simulink model "VxSpdEsti0725"  (R2022b)
settings: Solver=VariableStepAuto  StartTime=0.0  StopTime=10.0  RelTol=1e-3
undefined symbols (not defined in the file): DiscIntNeverNeededParam, Ldwf, Ldwr, Q, Qa, R, Ra, thr1, thr2, thr3, thr4, thr5, TrqRquRate
libraries: simulink x45
settings Model: Creator=12045  LastModifiedBy=12045

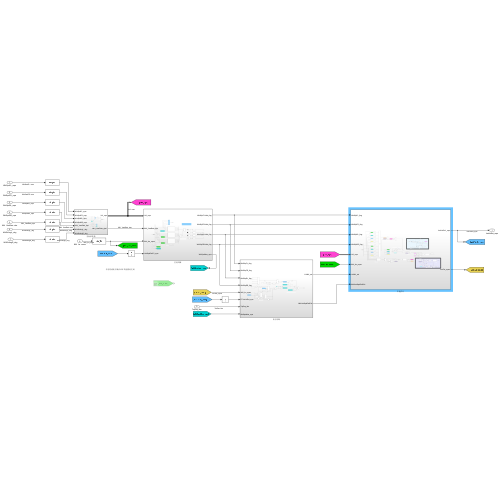
[thumbnail: Simulink's stored preview of the top-level diagram]
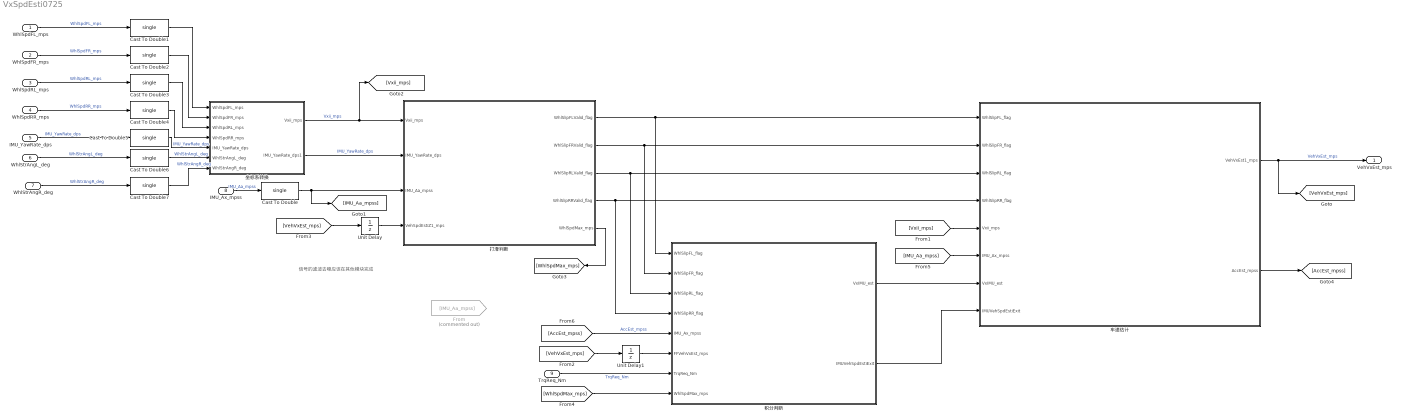
== system VxSpdEsti0725 ==
  note: 信号的滤波去噪应该在其他模块完成
  WhlSpdFL_mps : Inport
  WhlSpdFR_mps : Inport  Port=2
  WhlSpdRL_mps : Inport  Port=3
  WhlSpdRR_mps : Inport  Port=4
  IMU_YawRate_dps : Inport  Port=5
  WhlStrAngL_deg : Inport  Port=6
  WhlStrAngR_deg : Inport  Port=7
  IMU_Ax_mpss : Inport  Port=8
  TrqReq_Nm : Inport  Port=9
  Cast To Double{,1..7} (8 alike) : DataTypeConversion  OutDataTypeStr=single  SaturateOnIntegerOverflow=off  RndMeth=Floor
  From : From  Commented=on  GotoTag=IMU_Aa_mpss
  Unit Delay : UnitDelay  SampleTime=-1  HasFrameUpgradeWarning=on
  Unit Delay1 : UnitDelay  SampleTime=-1  HasFrameUpgradeWarning=on
  坐标系转换 : Subsystem
  打滑判断 : Subsystem
  积分判断 : Subsystem
  车速估计 : Subsystem
  VehVxEst_mps : Outport
  wires:
  [AccEst_mpss] -> 积分判断/5(IMU_Ax_mpss)  "AccEst_mpss"
  [Vxii_mps] -> 车速估计/5(Vxii_mps)
  Unit Delay/1 -> 打滑判断/4(VehSpdEstiZ1_mps)
  打滑判断/3(WhlSlipRLValid_flag) -> 积分判断/3(WhlSlipRL_flag), 车速估计/3(WhlSlipRL_flag)
  WhlSpdFR_mps/1 -> Cast To Double2/1  "WhlSpdFR_mps"
  打滑判断/5(WhlSpdMax_mps) -> [WhlSpdMax_mps]
  Cast To Double4/1 -> 坐标系转换/4(WhlSpdRR_mps)
  Cast To Double7/1 -> 坐标系转换/7(WhlStrAngR_deg)  "WhlStrAngR_deg"
  Unit Delay1/1 -> 积分判断/6(FFVehVxEst_mps)
  Cast To Double6/1 -> 坐标系转换/6(WhlStrAngL_deg)  "WhlStrAngL_deg"
  Cast To Double/1 -> [IMU_Aa_mpss], 打滑判断/3(IMU_Aa_mpss)
  Cast To Double3/1 -> 坐标系转换/3(WhlSpdRL_mps)
  WhlSpdFL_mps/1 -> Cast To Double1/1  "WhlSpdFL_mps"
  [VehVxEst_mps] -> Unit Delay/1
  TrqReq_Nm/1 -> 积分判断/7(TrqReq_Nm)  "TrqReq_Nm"
  [IMU_Aa_mpss] -> 车速估计/6(IMU_Ax_mpss)
  Cast To Double1/1 -> 坐标系转换/1(WhlSpdFL_mps)
  WhlSpdRR_mps/1 -> Cast To Double4/1  "WhlSpdRR_mps"
  打滑判断/2(WhlSlipFRValid_flag) -> 积分判断/2(WhlSlipFR_flag), 车速估计/2(WhlSlipFR_flag)
  Cast To Double2/1 -> 坐标系转换/2(WhlSpdFR_mps)
  [WhlSpdMax_mps] -> 积分判断/8(WhlSpdMax_mps)
  WhlSpdRL_mps/1 -> Cast To Double3/1  "WhlSpdRL_mps"
  车速估计/2(AccEst_mpss) -> [AccEst_mpss]
  积分判断/1(VxIMU_est) -> 车速估计/7(VxIMU_est)
  Cast To Double5/1 -> 坐标系转换/5(IMU_YawRate_dps)  "IMU_YawRate_dps"
  打滑判断/1(WhlSlipFLValid_flag) -> 积分判断/1(WhlSlipFL_flag), 车速估计/1(WhlSlipFL_flag)
  打滑判断/4(WhlSlipRRValid_flag) -> 积分判断/4(WhlSlipRR_flag), 车速估计/4(WhlSlipRR_flag)
  积分判断/2(IMUVehSpdEstiExit) -> 车速估计/8(IMUVehSpdEstiExit)
  [VehVxEst_mps] -> Unit Delay1/1
  IMU_Ax_mpss/1 -> Cast To Double/1  "IMU_Aa_mpss"
  WhlStrAngL_deg/1 -> Cast To Double6/1  "WhlStrAngL_deg"
  车速估计/1(VehVxEst1_mps) -> [VehVxEst_mps], VehVxEst_mps/1  "VehVxEst_mps"
  坐标系转换/2(IMU_YawRate_dps1) -> 打滑判断/2(IMU_YawRate_dps)  "IMU_YawRate_dps"
  IMU_YawRate_dps/1 -> Cast To Double5/1  "IMU_YawRate_dps"
  WhlStrAngR_deg/1 -> Cast To Double7/1  "WhlStrAngR_deg"
  坐标系转换/1(Vxii_mps) -> [Vxii_mps], 打滑判断/1(Vxii_mps)  "Vxii_mps"

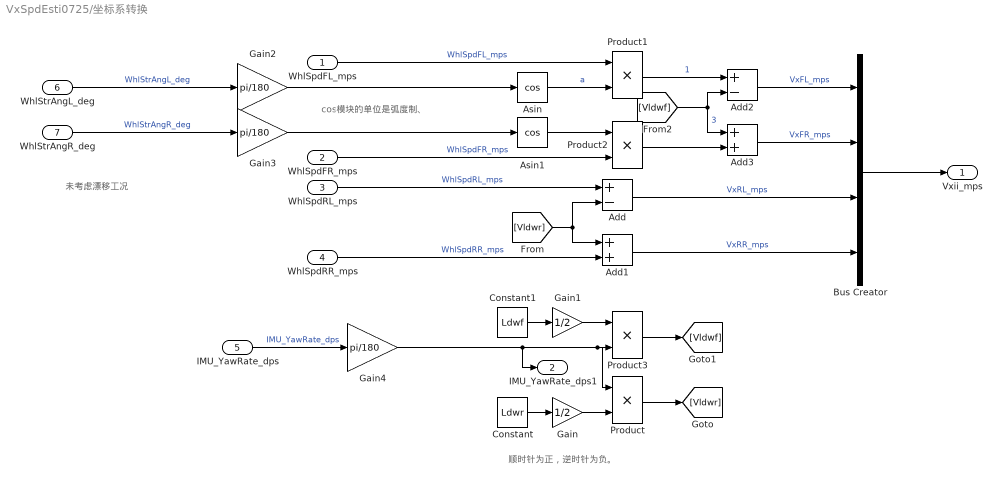
== system VxSpdEsti0725/坐标系转换 ==
  note: cos模块的单位是弧度制、
  note: 未考虑漂移工况
  note: 顺时针为正，逆时针为负。
  WhlSpdFL_mps : Inport
  WhlSpdFR_mps : Inport  Port=2
  WhlSpdRL_mps : Inport  Port=3
  WhlSpdRR_mps : Inport  Port=4
  IMU_YawRate_dps : Inport  Port=5
  WhlStrAngL_deg : Inport  Port=6
  WhlStrAngR_deg : Inport  Port=7
  Add : Sum  Inputs=+-
  Add1 : Sum
  Add2 : Sum  Inputs=+-
  Add3 : Sum
  Asin : Trigonometry  Operator=cos
  Asin1 : Trigonometry  Operator=cos
  Bus Creator : BusCreator  Inputs=4
  Constant : Constant  Value=Ldwr
  Constant1 : Constant  Value=Ldwf
  Gain : Gain  Gain=1/2
  Gain1 : Gain  Gain=1/2
  Gain2 : Gain  Gain=pi/180
  Gain3 : Gain  Gain=pi/180
  Gain4 : Gain  Gain=pi/180
  Product{,1..3} (4 alike) : Product
  Vxii_mps : Outport
  IMU_YawRate_dps1 : Outport  Port=2
  wires:
  Constant/1 -> Gain/1
  Gain/1 -> Product/2
  IMU_YawRate_dps/1 -> Gain4/1  "IMU_YawRate_dps"
  WhlSpdRL_mps/1 -> Add/1  "WhlSpdRL_mps"
  WhlSpdRR_mps/1 -> Add1/2  "WhlSpdRR_mps"
  Product/1 -> [Vldwr]
  [Vldwr] -> Add/2, Add1/1
  WhlSpdFL_mps/1 -> Product1/1  "WhlSpdFL_mps"
  WhlSpdFR_mps/1 -> Product2/2  "WhlSpdFR_mps"
  Constant1/1 -> Gain1/1
  Gain1/1 -> Product3/1
  Product3/1 -> [Vldwf]
  Product1/1 -> Add2/1  "1"
  [Vldwf] -> Add2/2, Add3/1  "3"
  Product2/1 -> Add3/2
  Add2/1 -> Bus Creator/1  "VxFL_mps"
  Add/1 -> Bus Creator/3  "VxRL_mps"
  Add3/1 -> Bus Creator/2  "VxFR_mps"
  Add1/1 -> Bus Creator/4  "VxRR_mps"
  Bus Creator/1 -> Vxii_mps/1
  Asin1/1 -> Product2/1
  WhlStrAngR_deg/1 -> Gain3/1  "WhlStrAngR_deg"
  WhlStrAngL_deg/1 -> Gain2/1  "WhlStrAngL_deg"
  Asin/1 -> Product1/2  "a"
  Gain2/1 -> Asin/1
  Gain3/1 -> Asin1/1
  Gain4/1 -> IMU_YawRate_dps1/1, Product/1, Product3/2

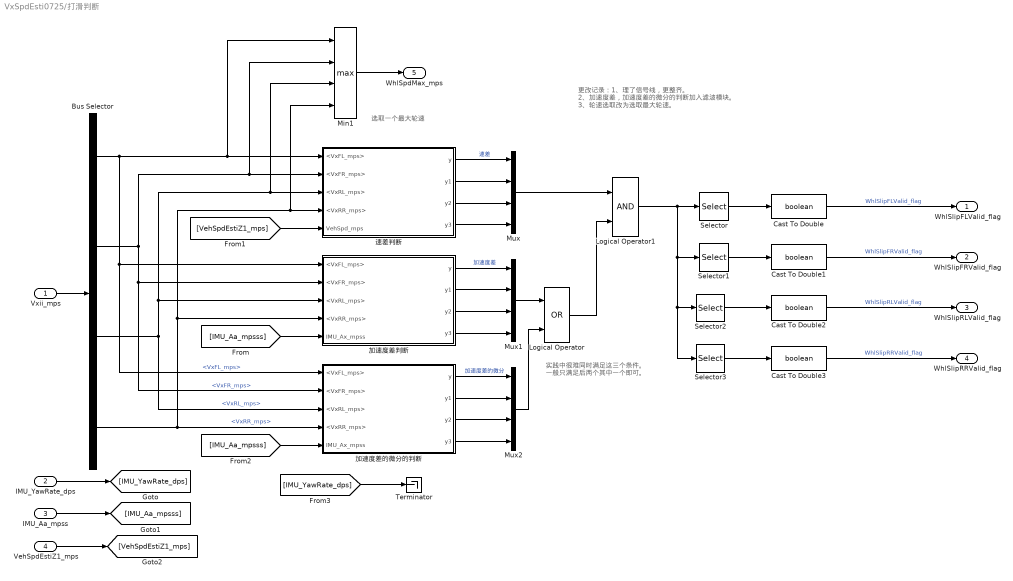
== system VxSpdEsti0725/打滑判断 ==
  note: 实践中很难同时满足这三个条件。
      | 一般只满足后两个其中一个即可。
  note: 更改记录：1、理了信号线，更整齐。
      | 2、加速度差，加速度差的微分的判断加入滤波模块。
      | 3、轮速选取改为选取最大轮速。
  note: 选取一个最大轮速
  Vxii_mps : Inport
  IMU_YawRate_dps : Inport  Port=2
  IMU_Aa_mpss : Inport  Port=3
  VehSpdEstiZ1_mps : Inport  Port=4
  Bus Selector : BusSelector  OutputSignals=VxFL_mps,VxFR_mps,VxRL_mps,VxRR_mps
  Cast To Double{,1..3} (4 alike) : DataTypeConversion  OutDataTypeStr=boolean  SaturateOnIntegerOverflow=off  RndMeth=Floor
  Logical Operator : Logic  Operator=OR  AllPortsSameDT=off  OutDataTypeStr=boolean
  Logical Operator1 : Logic  AllPortsSameDT=off  OutDataTypeStr=boolean
  Min1 : MinMax  Function=max  Inputs=4
  Mux : Mux
  Mux1 : Mux
  Mux2 : Mux
  Selector : Selector  InputPortWidth=4  IndexOptions=Index vector (dialog)  Indices=[1]  OutputSizes=1
  Selector1 : Selector  InputPortWidth=4  IndexOptions=Index vector (dialog)  Indices=[2]  OutputSizes=1
  Selector2 : Selector  InputPortWidth=4  IndexOptions=Index vector (dialog)  Indices=[3]  OutputSizes=1
  Selector3 : Selector  InputPortWidth=4  IndexOptions=Index vector (dialog)  Indices=[4]  OutputSizes=1
  Terminator : Terminator
  加速度差判断 : Subsystem
  加速度差的微分的判断 : Subsystem
  速差判断 : Subsystem
  WhlSlipFLValid_flag : Outport
  WhlSlipFRValid_flag : Outport  Port=2
  WhlSlipRLValid_flag : Outport  Port=3
  WhlSlipRRValid_flag : Outport  Port=4
  WhlSpdMax_mps : Outport  Port=5
  wires:
  Selector3/1 -> Cast To Double3/1
  Selector2/1 -> Cast To Double2/1
  [IMU_Aa_mpsss] -> 加速度差的微分的判断/5(IMU_Ax_mpss)
  [VehSpdEstiZ1_mps] -> 速差判断/5(VehSpd_mps)
  Bus Selector/3 -> 加速度差的微分的判断/3(<VxRL_mps>), 速差判断/3(<VxRL_mps>), Min1/3, 加速度差判断/3(<VxRL_mps>)  "<VxRL_mps>"
  Selector1/1 -> Cast To Double1/1
  [IMU_Aa_mpsss] -> 加速度差判断/5(IMU_Ax_mpss)
  Bus Selector/4 -> 加速度差判断/4(<VxRR_mps>), Min1/4, 速差判断/4(<VxRR_mps>), 加速度差的微分的判断/4(<VxRR_mps>)  "<VxRR_mps>"
  IMU_YawRate_dps/1 -> [IMU_YawRate_dps]
  Vxii_mps/1 -> Bus Selector/1
  Bus Selector/1 -> 加速度差的微分的判断/1(<VxFL_mps>), 加速度差判断/1(<VxFL_mps>), 速差判断/1(<VxFL_mps>), Min1/1  "<VxFL_mps>"
  VehSpdEstiZ1_mps/1 -> [VehSpdEstiZ1_mps]
  Selector/1 -> Cast To Double/1
  Bus Selector/2 -> 加速度差的微分的判断/2(<VxFR_mps>), 加速度差判断/2(<VxFR_mps>), 速差判断/2(<VxFR_mps>), Min1/2  "<VxFR_mps>"
  IMU_Aa_mpss/1 -> [IMU_Aa_mpsss]
  [IMU_YawRate_dps] -> Terminator/1
  Cast To Double/1 -> WhlSlipFLValid_flag/1  "WhlSlipFLValid_flag"
  Cast To Double1/1 -> WhlSlipFRValid_flag/1  "WhlSlipFRValid_flag"
  Cast To Double2/1 -> WhlSlipRLValid_flag/1  "WhlSlipRLValid_flag"
  Cast To Double3/1 -> WhlSlipRRValid_flag/1  "WhlSlipRRValid_flag"
  速差判断/1(y) -> Mux/1  "速差"
  速差判断/2(y1) -> Mux/2
  速差判断/3(y2) -> Mux/3
  速差判断/4(y3) -> Mux/4
  加速度差判断/1(y) -> Mux1/1  "加速度差"
  加速度差判断/2(y1) -> Mux1/2
  加速度差判断/3(y2) -> Mux1/3
  加速度差判断/4(y3) -> Mux1/4
  加速度差的微分的判断/1(y) -> Mux2/1  "加速度差的微分"
  加速度差的微分的判断/2(y1) -> Mux2/2
  加速度差的微分的判断/3(y2) -> Mux2/3
  加速度差的微分的判断/4(y3) -> Mux2/4
  Mux1/1 -> Logical Operator/1
  Mux2/1 -> Logical Operator/2
  Mux/1 -> Logical Operator1/1
  Logical Operator/1 -> Logical Operator1/2
  Logical Operator1/1 -> Selector3/1, Selector2/1, Selector1/1, Selector/1
  Min1/1 -> WhlSpdMax_mps/1

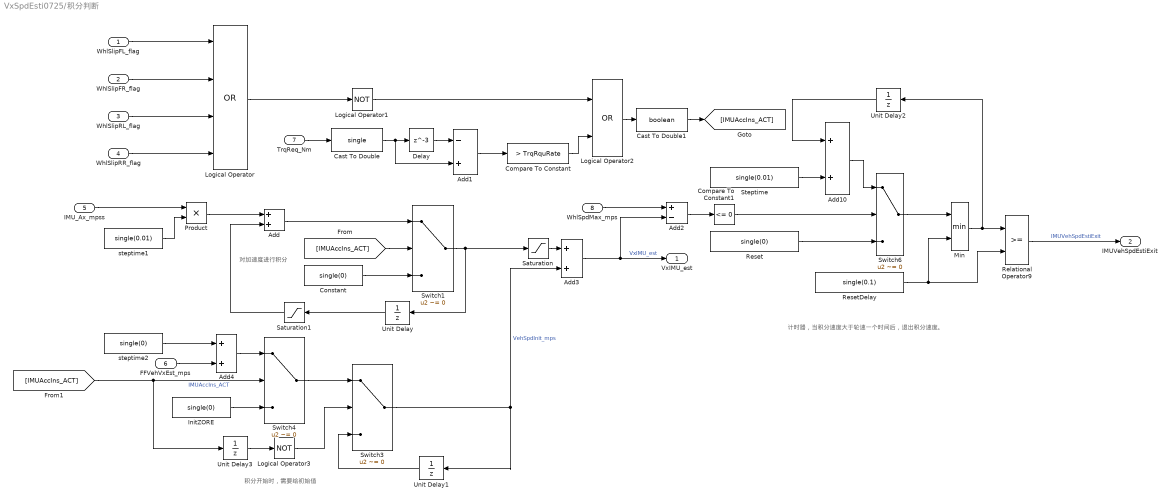
== system VxSpdEsti0725/积分判断 ==
  note: 对加速度进行积分
  note: 计时器，当积分速度大于轮速一个时间后，退出积分速度。
  note: 积分开始时，需要给初始值
  WhlSlipFL_flag : Inport
  WhlSlipFR_flag : Inport  Port=2
  WhlSlipRL_flag : Inport  Port=3
  WhlSlipRR_flag : Inport  Port=4
  IMU_Ax_mpss : Inport  Port=5
  FFVehVxEst_mps : Inport  Port=6
  TrqReq_Nm : Inport  Port=7
  WhlSpdMax_mps : Inport  Port=8
  Add{,3..4,10} (4 alike) : Sum
  Add1 : Sum  Inputs=-+
  Add2 : Sum  Inputs=+-
  Cast To Double : DataTypeConversion  OutDataTypeStr=single  SaturateOnIntegerOverflow=off  RndMeth=Floor
  Cast To Double1 : DataTypeConversion  OutDataTypeStr=boolean  SaturateOnIntegerOverflow=off  RndMeth=Floor
  Compare To Constant : simulink/Logic and Bit Operations/Compare To Constant  relop=>  const=TrqRquRate  OutDataTypeStr=boolean
  Compare To Constant1 : simulink/Logic and Bit Operations/Compare To Constant  relop=<=  const=0  OutDataTypeStr=boolean
  Constant : Constant  Value=single(0)
  Delay : Delay  DelayLength=3
  InitZORE : Constant  Value=single(0)
  Logical Operator : Logic  Operator=OR  Inputs=4  AllPortsSameDT=off  OutDataTypeStr=boolean
  Logical Operator1 : Logic  Operator=NOT  AllPortsSameDT=off  OutDataTypeStr=boolean
  Logical Operator2 : Logic  Operator=OR  AllPortsSameDT=off  OutDataTypeStr=boolean
  Logical Operator3 : Logic  Operator=NOT  AllPortsSameDT=off  OutDataTypeStr=boolean
  Min : MinMax  Inputs=2
  Product : Product
  Relational Operator9 : RelationalOperator  OutDataTypeStr=boolean  RndMeth=Simplest  InputSameDT=off
  Reset : Constant  Value=single(0)
  ResetDelay : Constant  Value=single(0.1)
  Saturation : Saturate  UpperLimit=200  LowerLimit=-10
  Saturation1 : Saturate  UpperLimit=200  LowerLimit=-10
  Steptime : Constant  Value=single(0.01)
  Switch{1,3..4,6} (4 alike) : Switch  Criteria=u2 ~= 0  SaturateOnIntegerOverflow=off  InputSameDT=off
  Unit Delay{,1..3} (4 alike) : UnitDelay  SampleTime=-1  HasFrameUpgradeWarning=on
  steptime1 : Constant  Value=single(0.01)
  steptime2 : Constant  Value=single(0)
  VxIMU_est : Outport
  IMUVehSpdEstiExit : Outport  Port=2
  wires:
  WhlSlipFL_flag/1 -> Logical Operator/1
  WhlSlipFR_flag/1 -> Logical Operator/2
  WhlSlipRL_flag/1 -> Logical Operator/3
  WhlSlipRR_flag/1 -> Logical Operator/4
  Logical Operator/1 -> Logical Operator1/1
  Unit Delay/1 -> Saturation1/1
  Add/1 -> Switch1/1
  Constant/1 -> Switch1/3
  Logical Operator1/1 -> Logical Operator2/1
  TrqReq_Nm/1 -> Cast To Double/1
  Delay/1 -> Add1/1
  Add1/1 -> Compare To Constant/1
  Compare To Constant/1 -> Logical Operator2/2
  [IMUAccIns_ACT] -> Switch1/2
  Logical Operator2/1 -> Cast To Double1/1
  Add2/1 -> Compare To Constant1/1
  WhlSpdMax_mps/1 -> Add2/1
  Saturation1/1 -> Add/2
  Product/1 -> Add/1
  IMU_Ax_mpss/1 -> Product/1
  steptime1/1 -> Product/2
  Saturation/1 -> Add3/1
  Add3/1 -> Add2/2, VxIMU_est/1  "VxIMU_est"
  Switch6/1 -> Min/1
  ResetDelay/1 -> Relational Operator9/2, Min/2
  Compare To Constant1/1 -> Switch6/2
  Add10/1 -> Switch6/1
  Steptime/1 -> Add10/2
  Min/1 -> Relational Operator9/1, Unit Delay2/1
  Reset/1 -> Switch6/3
  Unit Delay2/1 -> Add10/1
  Unit Delay3/1 -> Logical Operator3/1
  InitZORE/1 -> Switch4/3
  Logical Operator3/1 -> Switch3/2
  Switch3/1 -> Add3/2, Unit Delay1/1  "VehSpdInit_mps"
  Switch4/1 -> Switch3/1
  Cast To Double/1 -> Delay/1, Add1/2
  [IMUAccIns_ACT] -> Unit Delay3/1, Switch4/2  "IMUAccIns_ACT"
  Relational Operator9/1 -> IMUVehSpdEstiExit/1  "IMUVehSpdEstiExit"
  Cast To Double1/1 -> [IMUAccIns_ACT]
  Unit Delay1/1 -> Switch3/3
  Add4/1 -> Switch4/1
  FFVehVxEst_mps/1 -> Add4/2
  steptime2/1 -> Add4/1
  Switch1/1 -> Saturation/1, Unit Delay/1

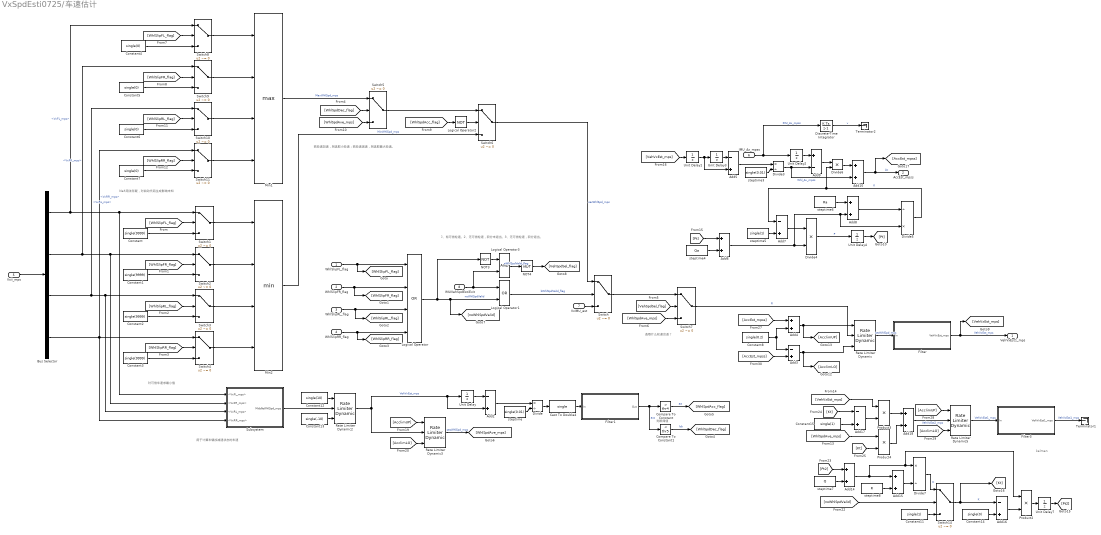
== system VxSpdEsti0725/车速估计 ==
  note: kalman
  note: 用于计算车辆加减速状态的车速
  note: 1、有可信轮速。2、无可信轮速，积分未退出。3、无可信轮速，积分退出。
  note: 选取什么轮速合适？
  note: 判断阈值
  note: 若轮速加速，则选取小轮速；若轮速减速，则选取最大轮速。
  note: NaN用法存疑，对自动代码生成影响未知
  note: 对可信车速求最小值
  WhlSlipFL_flag : Inport
  WhlSlipFR_flag : Inport  Port=2
  WhlSlipRL_flag : Inport  Port=3
  WhlSlipRR_flag : Inport  Port=4
  Vxii_mps : Inport  Port=5
  IMU_Ax_mpss : Inport  Port=6
  VxIMU_est : Inport  Port=7
  IMUVehSpdEstiExit : Inport  Port=8
  Add{4,6,8,10,14..15,18} (7 alike) : Sum
  Add{2..3,5,7,16..17} (6 alike) : Sum  Inputs=-+
  Add9 : Sum  Inputs=+-
  Bus Selector : BusSelector  OutputSignals=VxFL_mps,VxFR_mps,VxRL_mps,VxRR_mps
  Cast To Double4 : DataTypeConversion  OutDataTypeStr=single  SaturateOnIntegerOverflow=off  RndMeth=Floor
  Compare To Constant : simulink/Logic and Bit Operations/Compare To Constant  relop=>  const=thr4  OutDataTypeStr=boolean
  Compare To Constant1 : simulink/Logic and Bit Operations/Compare To Constant  relop=<  const=thr5  OutDataTypeStr=boolean
  Constant{,1..3} (4 alike) : Constant  Value=single(9999)
  Constant11 : Constant  Value=single(1)
  Constant12 : Constant  Value=single(10)
  Constant13 : Constant  Value=single(-10)
  Constant{4..7,14} (5 alike) : Constant  Value=single(0)
  Constant15 : Constant  Value=single(1)
  Constant8 : Constant  Value=single(0.2)
  Discrete-Time Integrator : DiscreteIntegrator  SampleTime=-1  ICPrevOutput=DiscIntNeverNeededParam  ICPrevScaledInput=DiscIntNeverNeededParam
  Divide : Product  Inputs=*/
  Divide3 : Product  Inputs=*/
  Divide4 : Product  Inputs=**
  Divide5 : Product  Inputs=/*
  Divide6 : Product  Inputs=**
  Divide7 : Product  Inputs=*/
  Filter : Subsystem
  Filter1 : Subsystem
  Filter3 : Subsystem
  Logical Operator : Logic  Operator=OR  Inputs=4  AllPortsSameDT=off  OutDataTypeStr=boolean
  Logical Operator1 : Logic  Operator=OR  AllPortsSameDT=off  OutDataTypeStr=boolean
  Logical Operator2 : Logic  Operator=NOT  AllPortsSameDT=off  OutDataTypeStr=boolean
  Logical Operator3 : Logic  AllPortsSameDT=off  OutDataTypeStr=boolean
  Min1 : MinMax  Function=max  Inputs=4
  Min2 : MinMax  Inputs=4
  NOT3 : Logic  Operator=NOT  AllPortsSameDT=off  OutDataTypeStr=boolean
  NOT4 : Logic  Operator=NOT  AllPortsSameDT=off  OutDataTypeStr=boolean
  Product2 : Product
  Product3 : Product
  Product4 : Product
  Rate Limiter Dynamic{,2..3,5} (4 alike) : simulink/Discontinuities/Rate Limiter Dynamic
  Subsystem : Subsystem
  Switch{,1..11,14} (13 alike) : Switch  Criteria=u2 ~= 0  SaturateOnIntegerOverflow=off  InputSameDT=off
  Terminator1 : Terminator
  Terminator2 : Terminator
  Unit Delay{,1..3,7} (5 alike) : UnitDelay  SampleTime=-1  HasFrameUpgradeWarning=on
  Unit Delay4 : UnitDelay  InitialCondition=0.01  SampleTime=-1  HasFrameUpgradeWarning=on
  steptime : Constant  Value=single(0.01)
  steptime3 : Constant  Value=single(0.01)
  steptime4 : Constant  Value=Qa
  steptime5 : Constant  Value=single(1)
  steptime6 : Constant  Value=Ra
  steptime7 : Constant  Value=Q
  steptime8 : Constant  Value=R
  VehVxEst1_mps : Outport
  AccEst_mpss : Outport  Port=2
  wires:
  Compare To Constant/1 -> [WhlSpdAcc_flag]  "aa"
  Vxii_mps/1 -> Bus Selector/1
  WhlSlipRR_flag/1 -> [WhlSlipRR_flag], Logical Operator/4
  Logical Operator3/1 -> NOT4/1  "aWhlSpdValid_flag"
  [VehSpdSel_flag] -> Switch7/2
  Logical Operator2/1 -> Switch6/2
  [WhlSlipFL_flag] -> Switch1/2
  Switch5/1 -> Switch6/1
  Constant/1 -> Switch1/3
  Compare To Constant1/1 -> [WhlSpdDec_flag]  "bb"
  Unit Delay/1 -> Add2/1
  [WhlSpdAve_mps] -> Switch5/3
  Filter1/1(Out) -> Compare To Constant1/1, Compare To Constant/1  "acc"
  Constant3/1 -> Switch4/3
  Logical Operator1/1 -> Switch/2  "bWhlSpdValid_flag"
  Switch4/1 -> Min2/4
  Constant2/1 -> Switch3/3
  [WhlSlipRR_flag] -> Switch4/2
  Switch1/1 -> Min2/1
  WhlSlipFR_flag/1 -> [WhlSlipFR_flag], Logical Operator/2
  [WhlSpdAcc_flag] -> Logical Operator2/1
  [WhlSlipRL_flag] -> Switch3/2
  Switch2/1 -> Min2/2
  Logical Operator/1 -> [noWhlSpdValid], Logical Operator1/2, NOT3/1  "noWhlSpdValid"
  WhlSlipFL_flag/1 -> [WhlSlipFL_flag], Logical Operator/1
  Constant1/1 -> Switch2/3
  Cast To Double4/1 -> Filter1/1(In)
  [WhlSpdDec_flag] -> Switch5/2
  [WhlSlipFR_flag] -> Switch2/2
  WhlSlipRL_flag/1 -> [WhlSlipRL_flag], Logical Operator/3
  Switch3/1 -> Min2/3
  [WhlSpdAve_mps] -> Switch7/3
  Add2/1 -> Divide/1
  Divide/1 -> Cast To Double4/1
  steptime/1 -> Divide/2
  Bus Selector/1 -> Switch8/1, Subsystem/1(<VxFL_mps>), Switch1/1  "<VxFL_mps>"
  Bus Selector/4 -> Subsystem/4(<VxRR_mps>), Switch11/1, Switch4/1  "<VxRR_mps>"
  [WhlSlipFR_flag] -> Switch9/2
  Bus Selector/2 -> Switch9/1, Subsystem/2(<VxFR_mps>), Switch2/1  "<VxFR_mps>"
  Constant5/1 -> Switch9/3
  Bus Selector/3 -> Switch10/1, Subsystem/3(<VxRL_mps>), Switch3/1  "<VxRL_mps>"
  [WhlSlipRL_flag] -> Switch10/2
  [WhlSlipRR_flag] -> Switch11/2
  Constant6/1 -> Switch10/3
  Constant7/1 -> Switch11/3
  Constant4/1 -> Switch8/3
  [WhlSlipFL_flag] -> Switch8/2
  Switch8/1 -> Min1/1
  Switch9/1 -> Min1/2
  Switch10/1 -> Min1/3
  Switch11/1 -> Min1/4
  Min1/1 -> Switch5/1  "MaxWhlSpd_mps"
  Subsystem/1(MiddleWhlSpd_mps) -> Rate Limiter Dynamic2/2
  Constant12/1 -> Rate Limiter Dynamic2/1
  Constant13/1 -> Rate Limiter Dynamic2/3
  Rate Limiter Dynamic2/1 -> Rate Limiter Dynamic3/2, Add2/2, Unit Delay/1  "VehVxEst_mps"
  Min2/1 -> Switch6/3  "MinWhlSpd_mps"
  IMUVehSpdEstiExit/1 -> Logical Operator3/2, Logical Operator1/1
  NOT3/1 -> Logical Operator3/1
  NOT4/1 -> [VehSpdSel_flag]
  Divide5/1 -> Add7/1, Divide6/2  "K"
  Unit Delay3/1 -> Add5/1
  steptime3/1 -> Divide3/2
  Add5/1 -> Divide3/1
  Unit Delay4/1 -> [Pt]
  [Pt] -> Add6/1
  steptime4/1 -> Add6/2
  Add6/1 -> Divide5/2, Add8/2, Divide4/2
  steptime5/1 -> Add7/2
  Add7/1 -> Divide4/1
  Divide4/1 -> Unit Delay4/1  "P"
  steptime6/1 -> Add8/1
  Add8/1 -> Divide5/1
  Divide3/1 -> Add10/2, Add9/2  "Whl_Ax_mpss"
  Add9/1 -> Divide6/1
  Divide6/1 -> Add10/1
  Add10/1 -> AccEst_mpss/1, [AccEst_mpss]  "Ax"
  IMU_Ax_mpss/1 -> Unit Delay2/1, Discrete-Time Integrator/1  "IMU_Ax_mpss"
  VxIMU_est/1 -> Switch/3
  Rate Limiter Dynamic3/1 -> [WhlSpdAve_mps]  "secWhlSpd_mps"
  [AcclimUP] -> Rate Limiter Dynamic3/1
  [AcclimLO] -> Rate Limiter Dynamic3/3
  Filter/1(VehVxEst_mps) -> [VehVxEst_mps], VehVxEst1_mps/1  "VehVxEst_mps"
  Unit Delay7/1 -> [Pt2]
  Add14/1 -> Add15/1, Product2/1, Divide7/1
  steptime7/1 -> Add14/2
  steptime8/1 -> Add15/2
  Add15/1 -> Divide7/2
  Switch14/1 -> [Kt], Add16/1  "K"
  Constant14/1 -> Add16/2
  Add16/1 -> Product2/2
  Product2/1 -> Unit Delay7/1
  [Pt2] -> Add14/1
  Constant15/1 -> Add17/2
  [Kt] -> Add17/1
  Add17/1 -> Product3/2
  Product3/1 -> Add18/1
  [Kt] -> Product4/2
  Product4/1 -> Add18/2
  Switch/1 -> Switch7/1
  Divide7/1 -> Switch14/1  "K"
  Constant11/1 -> Switch14/3
  Add18/1 -> Rate Limiter Dynamic5/2  "VehVxEst2_mps"
  Rate Limiter Dynamic5/1 -> Filter3/1(In)  "VehVxEst1_mps"
  [AcclimUP] -> Rate Limiter Dynamic5/1
  [AcclimLO] -> Rate Limiter Dynamic5/3
  Discrete-Time Integrator/1 -> Terminator2/1  "v"
  [noWhlSpdValid] -> Switch14/2
  [AccEst_mpss] -> Add4/1
  [AccEst_mpss] -> Add3/2
  Filter3/1(VehVxEst1_mps) -> Terminator1/1  "VehVxEst1_mps"
  [VehVxEst_mps] -> Unit Delay1/1
  Unit Delay2/1 -> Add9/1
  Switch6/1 -> Switch/1  "secWhlSpd_mps"
  Constant8/1 -> Add3/1, Add4/2
  Add4/1 -> [AcclimUP], Rate Limiter Dynamic/1
  Add3/1 -> [AcclimLO], Rate Limiter Dynamic/3
  Switch7/1 -> Rate Limiter Dynamic/2  "R"
  Rate Limiter Dynamic/1 -> Filter/1(In)  "secWhlSpd_mps"
  [WhlSpdAve_mps] -> Product4/1
  [VehVxEst_mps] -> Product3/1
  Unit Delay1/1 -> Add5/2, Unit Delay3/1

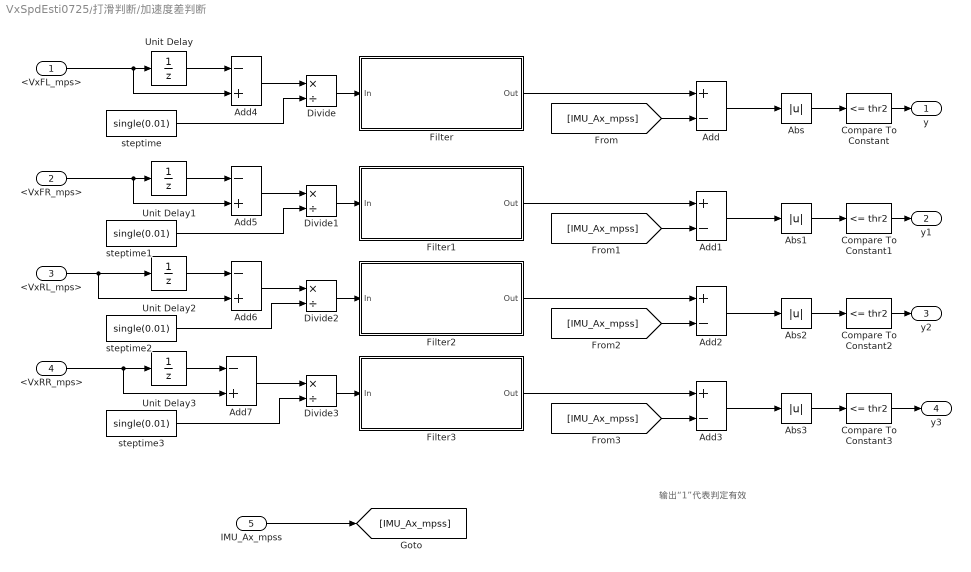
== system VxSpdEsti0725/打滑判断/加速度差判断 ==
  note: 输出“1”代表判定有效
  <VxFL_mps> : Inport
  <VxFR_mps> : Inport  Port=2
  <VxRL_mps> : Inport  Port=3
  <VxRR_mps> : Inport  Port=4
  IMU_Ax_mpss : Inport  Port=5
  Abs{,1..3} (4 alike) : Abs  SaturateOnIntegerOverflow=off
  Add{,1..3} (4 alike) : Sum  Inputs=+-
  Add{4..7} (4 alike) : Sum  Inputs=-+
  Compare To Constant{,1..3} (4 alike) : simulink/Logic and Bit Operations/Compare To Constant  relop=<=  const=thr2  OutDataTypeStr=boolean
  Divide{,1..3} (4 alike) : Product  Inputs=*/
  Filter : Subsystem
  Filter1 : Subsystem
  Filter2 : Subsystem
  Filter3 : Subsystem
  Unit Delay{,1..3} (4 alike) : UnitDelay  SampleTime=-1  HasFrameUpgradeWarning=on
  steptime{,1..3} (4 alike) : Constant  Value=single(0.01)
  y : Outport
  y1 : Outport  Port=2
  y2 : Outport  Port=3
  y3 : Outport  Port=4
  wires:
  Compare To Constant/1 -> y/1
  Compare To Constant2/1 -> y2/1
  Abs2/1 -> Compare To Constant2/1
  Add1/1 -> Abs1/1
  Abs/1 -> Compare To Constant/1
  [IMU_Ax_mpss] -> Add3/2
  [IMU_Ax_mpss] -> Add2/2
  [IMU_Ax_mpss] -> Add/2
  Abs3/1 -> Compare To Constant3/1
  Compare To Constant3/1 -> y3/1
  Compare To Constant1/1 -> y1/1
  [IMU_Ax_mpss] -> Add1/2
  Add/1 -> Abs/1
  Add3/1 -> Abs3/1
  Abs1/1 -> Compare To Constant1/1
  Add2/1 -> Abs2/1
  <VxFL_mps>/1 -> Add4/2, Unit Delay/1
  Unit Delay/1 -> Add4/1
  Add4/1 -> Divide/1
  steptime/1 -> Divide/2
  Divide/1 -> Filter/1(In)
  IMU_Ax_mpss/1 -> [IMU_Ax_mpss]
  steptime1/1 -> Divide1/2
  Add5/1 -> Divide1/1
  Unit Delay1/1 -> Add5/1
  <VxFR_mps>/1 -> Unit Delay1/1, Add5/2
  Divide1/1 -> Filter1/1(In)
  steptime2/1 -> Divide2/2
  Add6/1 -> Divide2/1
  Unit Delay2/1 -> Add6/1
  <VxRL_mps>/1 -> Unit Delay2/1, Add6/2
  Divide2/1 -> Filter2/1(In)
  steptime3/1 -> Divide3/2
  Add7/1 -> Divide3/1
  Unit Delay3/1 -> Add7/1
  <VxRR_mps>/1 -> Unit Delay3/1, Add7/2
  Divide3/1 -> Filter3/1(In)
  Filter/1(Out) -> Add/1
  Filter1/1(Out) -> Add1/1
  Filter2/1(Out) -> Add2/1
  Filter3/1(Out) -> Add3/1

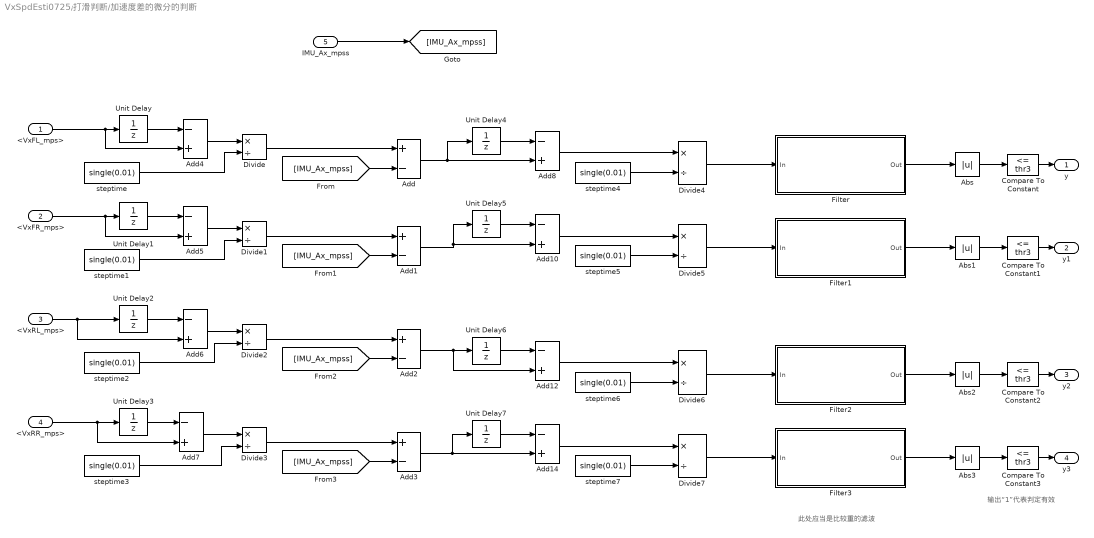
== system VxSpdEsti0725/打滑判断/加速度差的微分的判断 ==
  note: 此处应当是比较重的滤波
  note: 输出“1”代表判定有效
  <VxFL_mps> : Inport
  <VxFR_mps> : Inport  Port=2
  <VxRL_mps> : Inport  Port=3
  <VxRR_mps> : Inport  Port=4
  IMU_Ax_mpss : Inport  Port=5
  Abs{,1..3} (4 alike) : Abs  SaturateOnIntegerOverflow=off
  Add{,1..3} (4 alike) : Sum  Inputs=+-
  Add{4..8,10,12,14} (8 alike) : Sum  Inputs=-+
  Compare To Constant{,1..3} (4 alike) : simulink/Logic and Bit Operations/Compare To Constant  relop=<=  const=thr3  OutDataTypeStr=boolean
  Divide{,1..7} (8 alike) : Product  Inputs=*/
  Filter : Subsystem
  Filter1 : Subsystem
  Filter2 : Subsystem
  Filter3 : Subsystem
  Unit Delay{,1..7} (8 alike) : UnitDelay  SampleTime=-1  HasFrameUpgradeWarning=on
  steptime{,1..7} (8 alike) : Constant  Value=single(0.01)
  y : Outport
  y1 : Outport  Port=2
  y2 : Outport  Port=3
  y3 : Outport  Port=4
  wires:
  Divide3/1 -> Add3/1
  <VxRR_mps>/1 -> Add7/2, Unit Delay3/1
  Unit Delay3/1 -> Add7/1
  Add7/1 -> Divide3/1
  steptime3/1 -> Divide3/2
  Divide2/1 -> Add2/1
  <VxRL_mps>/1 -> Add6/2, Unit Delay2/1
  Unit Delay2/1 -> Add6/1
  Add6/1 -> Divide2/1
  steptime2/1 -> Divide2/2
  Divide1/1 -> Add1/1
  <VxFR_mps>/1 -> Add5/2, Unit Delay1/1
  Unit Delay1/1 -> Add5/1
  Add5/1 -> Divide1/1
  steptime1/1 -> Divide1/2
  IMU_Ax_mpss/1 -> [IMU_Ax_mpss]
  Divide/1 -> Add/1
  steptime/1 -> Divide/2
  Add4/1 -> Divide/1
  Unit Delay/1 -> Add4/1
  <VxFL_mps>/1 -> Unit Delay/1, Add4/2
  Abs1/1 -> Compare To Constant1/1
  [IMU_Ax_mpss] -> Add1/2
  Compare To Constant1/1 -> y1/1
  Compare To Constant3/1 -> y3/1
  Abs3/1 -> Compare To Constant3/1
  [IMU_Ax_mpss] -> Add/2
  [IMU_Ax_mpss] -> Add2/2
  [IMU_Ax_mpss] -> Add3/2
  Abs/1 -> Compare To Constant/1
  Abs2/1 -> Compare To Constant2/1
  Compare To Constant2/1 -> y2/1
  Compare To Constant/1 -> y/1
  Add/1 -> Add8/2, Unit Delay4/1
  Unit Delay4/1 -> Add8/1
  Add8/1 -> Divide4/1
  steptime4/1 -> Divide4/2
  Divide4/1 -> Filter/1(In)
  steptime5/1 -> Divide5/2
  Add10/1 -> Divide5/1
  Unit Delay5/1 -> Add10/1
  Add1/1 -> Unit Delay5/1, Add10/2
  Divide5/1 -> Filter1/1(In)
  Divide6/1 -> Filter2/1(In)
  Add2/1 -> Add12/2, Unit Delay6/1
  Add12/1 -> Divide6/1
  steptime6/1 -> Divide6/2
  Unit Delay6/1 -> Add12/1
  steptime7/1 -> Divide7/2
  Add14/1 -> Divide7/1
  Add3/1 -> Unit Delay7/1, Add14/2
  Unit Delay7/1 -> Add14/1
  Divide7/1 -> Filter3/1(In)
  Filter/1(Out) -> Abs/1
  Filter1/1(Out) -> Abs1/1
  Filter2/1(Out) -> Abs2/1
  Filter3/1(Out) -> Abs3/1

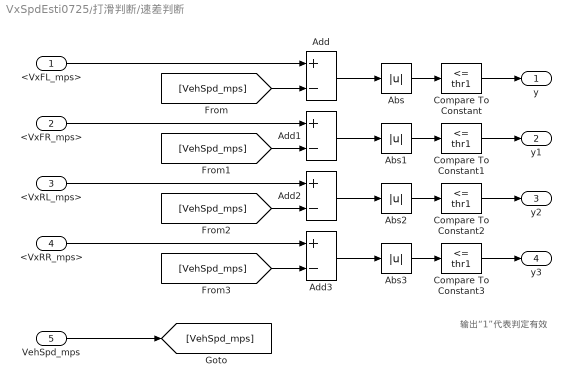
== system VxSpdEsti0725/打滑判断/速差判断 ==
  note: 输出“1”代表判定有效
  <VxFL_mps> : Inport
  <VxFR_mps> : Inport  Port=2
  <VxRL_mps> : Inport  Port=3
  <VxRR_mps> : Inport  Port=4
  VehSpd_mps : Inport  Port=5
  Abs{,1..3} (4 alike) : Abs  SaturateOnIntegerOverflow=off
  Add{,1..3} (4 alike) : Sum  Inputs=+-
  Compare To Constant{,1..3} (4 alike) : simulink/Logic and Bit Operations/Compare To Constant  relop=<=  const=thr1  OutDataTypeStr=boolean
  y : Outport
  y1 : Outport  Port=2
  y2 : Outport  Port=3
  y3 : Outport  Port=4
  wires:
  Add2/1 -> Abs2/1
  Abs1/1 -> Compare To Constant1/1
  <VxRR_mps>/1 -> Add3/1
  Add3/1 -> Abs3/1
  Add/1 -> Abs/1
  [VehSpd_mps] -> Add1/2
  <VxRL_mps>/1 -> Add2/1
  <VxFR_mps>/1 -> Add1/1
  Compare To Constant1/1 -> y1/1
  Compare To Constant3/1 -> y3/1
  Abs3/1 -> Compare To Constant3/1
  [VehSpd_mps] -> Add/2
  [VehSpd_mps] -> Add2/2
  [VehSpd_mps] -> Add3/2
  Abs/1 -> Compare To Constant/1
  Add1/1 -> Abs1/1
  Abs2/1 -> Compare To Constant2/1
  <VxFL_mps>/1 -> Add/1
  Compare To Constant2/1 -> y2/1
  Compare To Constant/1 -> y/1
  VehSpd_mps/1 -> [VehSpd_mps]

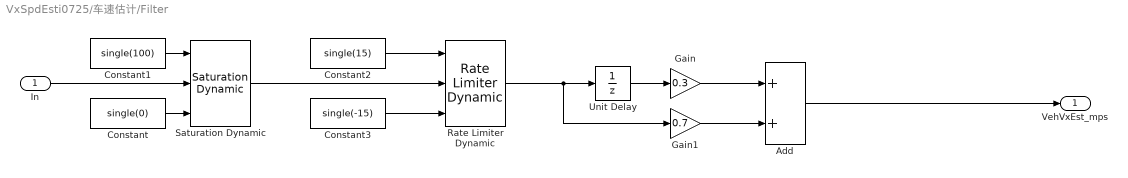
== system VxSpdEsti0725/车速估计/Filter ==
  In : Inport
  Add : Sum
  Constant : Constant  Value=single(0)
  Constant1 : Constant  Value=single(100)
  Constant2 : Constant  Value=single(15)
  Constant3 : Constant  Value=single(-15)
  Gain : Gain  Gain=0.3
  Gain1 : Gain  Gain=0.7
  Rate Limiter Dynamic : simulink/Discontinuities/Rate Limiter Dynamic
  Saturation Dynamic : simulink/Discontinuities/Saturation Dynamic  OutMin=[]  OutMax=[]  OutDataTypeStr=Inherit: Same as second input  OutDataType=fixdt(1, 16)  OutScaling=2^-10  DoSatur=off
  Unit Delay : UnitDelay  SampleTime=-1  HasFrameUpgradeWarning=on
  VehVxEst_mps : Outport
  wires:
  In/1 -> Saturation Dynamic/2
  Saturation Dynamic/1 -> Rate Limiter Dynamic/2
  Constant1/1 -> Saturation Dynamic/1
  Constant/1 -> Saturation Dynamic/3
  Unit Delay/1 -> Gain/1
  Gain/1 -> Add/1
  Gain1/1 -> Add/2
  Rate Limiter Dynamic/1 -> Gain1/1, Unit Delay/1
  Add/1 -> VehVxEst_mps/1
  Constant2/1 -> Rate Limiter Dynamic/1
  Constant3/1 -> Rate Limiter Dynamic/3

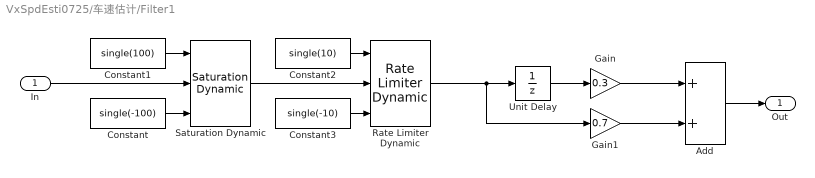
== system VxSpdEsti0725/车速估计/Filter1 ==
  In : Inport
  Add : Sum
  Constant : Constant  Value=single(-100)
  Constant1 : Constant  Value=single(100)
  Constant2 : Constant  Value=single(10)
  Constant3 : Constant  Value=single(-10)
  Gain : Gain  Gain=0.3
  Gain1 : Gain  Gain=0.7
  Rate Limiter Dynamic : simulink/Discontinuities/Rate Limiter Dynamic
  Saturation Dynamic : simulink/Discontinuities/Saturation Dynamic  OutMin=[]  OutMax=[]  OutDataTypeStr=Inherit: Same as second input  OutDataType=fixdt(1, 16)  OutScaling=2^-10  DoSatur=off
  Unit Delay : UnitDelay  SampleTime=-1  HasFrameUpgradeWarning=on
  Out : Outport
  wires:
  In/1 -> Saturation Dynamic/2
  Saturation Dynamic/1 -> Rate Limiter Dynamic/2
  Constant1/1 -> Saturation Dynamic/1
  Constant/1 -> Saturation Dynamic/3
  Constant2/1 -> Rate Limiter Dynamic/1
  Constant3/1 -> Rate Limiter Dynamic/3
  Unit Delay/1 -> Gain/1
  Gain/1 -> Add/1
  Add/1 -> Out/1
  Gain1/1 -> Add/2
  Rate Limiter Dynamic/1 -> Unit Delay/1, Gain1/1

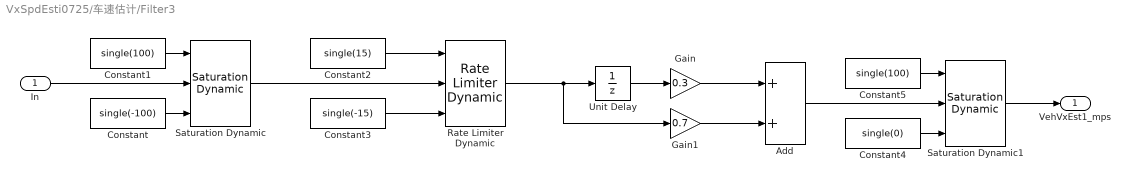
== system VxSpdEsti0725/车速估计/Filter3 ==
  In : Inport
  Add : Sum
  Constant : Constant  Value=single(-100)
  Constant1 : Constant  Value=single(100)
  Constant2 : Constant  Value=single(15)
  Constant3 : Constant  Value=single(-15)
  Constant4 : Constant  Value=single(0)
  Constant5 : Constant  Value=single(100)
  Gain : Gain  Gain=0.3
  Gain1 : Gain  Gain=0.7
  Rate Limiter Dynamic : simulink/Discontinuities/Rate Limiter Dynamic
  Saturation Dynamic : simulink/Discontinuities/Saturation Dynamic  OutMin=[]  OutMax=[]  OutDataTypeStr=Inherit: Same as second input  OutDataType=fixdt(1, 16)  OutScaling=2^-10  DoSatur=off
  Saturation Dynamic1 : simulink/Discontinuities/Saturation Dynamic  OutMin=[]  OutMax=[]  OutDataTypeStr=Inherit: Same as second input  OutDataType=fixdt(1, 16)  OutScaling=2^-10  DoSatur=off
  Unit Delay : UnitDelay  SampleTime=-1  HasFrameUpgradeWarning=on
  VehVxEst1_mps : Outport
  wires:
  Constant3/1 -> Rate Limiter Dynamic/3
  Constant2/1 -> Rate Limiter Dynamic/1
  Saturation Dynamic1/1 -> VehVxEst1_mps/1
  Add/1 -> Saturation Dynamic1/2
  Constant5/1 -> Saturation Dynamic1/1
  Constant4/1 -> Saturation Dynamic1/3
  Rate Limiter Dynamic/1 -> Unit Delay/1, Gain1/1
  Gain1/1 -> Add/2
  Gain/1 -> Add/1
  Unit Delay/1 -> Gain/1
  Constant/1 -> Saturation Dynamic/3
  Constant1/1 -> Saturation Dynamic/1
  Saturation Dynamic/1 -> Rate Limiter Dynamic/2
  In/1 -> Saturation Dynamic/2

== system VxSpdEsti0725/车速估计/Subsystem ==
  <VxFL_mps> : Inport
  <VxFR_mps> : Inport  Port=2
  <VxRL_mps> : Inport  Port=3
  <VxRR_mps> : Inport  Port=4
  Add3 : Sum  Inputs=++++
  Add4 : Sum  Inputs=+--
  Gain1 : Gain  Gain=1/2
  Min3 : MinMax  Function=max  Inputs=4
  Min4 : MinMax  Inputs=4
  Subsystem : Subsystem  Commented=on
  MiddleWhlSpd_mps : Outport
  wires:
  Add4/1 -> Gain1/1
  Add3/1 -> Add4/1
  Min3/1 -> Add4/3
  <VxRR_mps>/1 -> Min3/4, Add3/1, Min4/4
  <VxRL_mps>/1 -> Min3/3, Min4/3, Add3/2
  <VxFR_mps>/1 -> Min4/2, Min3/2, Add3/3
  Min4/1 -> Add4/2
  <VxFL_mps>/1 -> Add3/4, Min4/1, Min3/1
  Gain1/1 -> MiddleWhlSpd_mps/1  "MaxWhlSpd_mps"

== system VxSpdEsti0725/打滑判断/加速度差判断/Filter ==
  In : Inport
  Add : Sum
  Constant : Constant  Value=single(-100)
  Constant1 : Constant  Value=single(100)
  Constant2 : Constant  Value=single(100)
  Constant3 : Constant  Value=single(-100)
  Gain : Gain  Gain=0.3
  Gain1 : Gain  Gain=0.7
  Rate Limiter Dynamic : simulink/Discontinuities/Rate Limiter Dynamic
  Saturation Dynamic : simulink/Discontinuities/Saturation Dynamic  OutMin=[]  OutMax=[]  OutDataTypeStr=Inherit: Same as second input  OutDataType=fixdt(1, 16)  OutScaling=2^-10  DoSatur=off
  Unit Delay : UnitDelay  SampleTime=-1  HasFrameUpgradeWarning=on
  Out : Outport
  wires:
  In/1 -> Saturation Dynamic/2
  Saturation Dynamic/1 -> Rate Limiter Dynamic/2
  Constant1/1 -> Saturation Dynamic/1
  Constant/1 -> Saturation Dynamic/3
  Constant2/1 -> Rate Limiter Dynamic/1
  Constant3/1 -> Rate Limiter Dynamic/3
  Unit Delay/1 -> Gain/1
  Gain/1 -> Add/1
  Add/1 -> Out/1
  Gain1/1 -> Add/2
  Rate Limiter Dynamic/1 -> Gain1/1, Unit Delay/1

== system VxSpdEsti0725/打滑判断/加速度差判断/Filter1 ==
  In : Inport
  Add : Sum
  Constant : Constant  Value=single(-100)
  Constant1 : Constant  Value=single(100)
  Constant2 : Constant  Value=single(100)
  Constant3 : Constant  Value=single(-100)
  Gain : Gain  Gain=0.3
  Gain1 : Gain  Gain=0.7
  Rate Limiter Dynamic : simulink/Discontinuities/Rate Limiter Dynamic
  Saturation Dynamic : simulink/Discontinuities/Saturation Dynamic  OutMin=[]  OutMax=[]  OutDataTypeStr=Inherit: Same as second input  OutDataType=fixdt(1, 16)  OutScaling=2^-10  DoSatur=off
  Unit Delay : UnitDelay  SampleTime=-1  HasFrameUpgradeWarning=on
  Out : Outport
  wires:
  Rate Limiter Dynamic/1 -> Unit Delay/1, Gain1/1
  Gain1/1 -> Add/2
  Add/1 -> Out/1
  Gain/1 -> Add/1
  Unit Delay/1 -> Gain/1
  Constant3/1 -> Rate Limiter Dynamic/3
  Constant2/1 -> Rate Limiter Dynamic/1
  Constant/1 -> Saturation Dynamic/3
  Constant1/1 -> Saturation Dynamic/1
  Saturation Dynamic/1 -> Rate Limiter Dynamic/2
  In/1 -> Saturation Dynamic/2

== system VxSpdEsti0725/打滑判断/加速度差判断/Filter2 ==
  In : Inport
  Add : Sum
  Constant : Constant  Value=single(-100)
  Constant1 : Constant  Value=single(100)
  Constant2 : Constant  Value=single(100)
  Constant3 : Constant  Value=single(-100)
  Gain : Gain  Gain=0.3
  Gain1 : Gain  Gain=0.7
  Rate Limiter Dynamic : simulink/Discontinuities/Rate Limiter Dynamic
  Saturation Dynamic : simulink/Discontinuities/Saturation Dynamic  OutMin=[]  OutMax=[]  OutDataTypeStr=Inherit: Same as second input  OutDataType=fixdt(1, 16)  OutScaling=2^-10  DoSatur=off
  Unit Delay : UnitDelay  SampleTime=-1  HasFrameUpgradeWarning=on
  Out : Outport
  wires:
  In/1 -> Saturation Dynamic/2
  Saturation Dynamic/1 -> Rate Limiter Dynamic/2
  Constant1/1 -> Saturation Dynamic/1
  Constant/1 -> Saturation Dynamic/3
  Constant2/1 -> Rate Limiter Dynamic/1
  Constant3/1 -> Rate Limiter Dynamic/3
  Unit Delay/1 -> Gain/1
  Gain/1 -> Add/1
  Add/1 -> Out/1
  Gain1/1 -> Add/2
  Rate Limiter Dynamic/1 -> Gain1/1, Unit Delay/1

== system VxSpdEsti0725/打滑判断/加速度差判断/Filter3 ==
  In : Inport
  Add : Sum
  Constant : Constant  Value=single(-100)
  Constant1 : Constant  Value=single(100)
  Constant2 : Constant  Value=single(100)
  Constant3 : Constant  Value=single(-100)
  Gain : Gain  Gain=0.3
  Gain1 : Gain  Gain=0.7
  Rate Limiter Dynamic : simulink/Discontinuities/Rate Limiter Dynamic
  Saturation Dynamic : simulink/Discontinuities/Saturation Dynamic  OutMin=[]  OutMax=[]  OutDataTypeStr=Inherit: Same as second input  OutDataType=fixdt(1, 16)  OutScaling=2^-10  DoSatur=off
  Unit Delay : UnitDelay  SampleTime=-1  HasFrameUpgradeWarning=on
  Out : Outport
  wires:
  Rate Limiter Dynamic/1 -> Unit Delay/1, Gain1/1
  Gain1/1 -> Add/2
  Add/1 -> Out/1
  Gain/1 -> Add/1
  Unit Delay/1 -> Gain/1
  Constant3/1 -> Rate Limiter Dynamic/3
  Constant2/1 -> Rate Limiter Dynamic/1
  Constant/1 -> Saturation Dynamic/3
  Constant1/1 -> Saturation Dynamic/1
  Saturation Dynamic/1 -> Rate Limiter Dynamic/2
  In/1 -> Saturation Dynamic/2

== system VxSpdEsti0725/打滑判断/加速度差的微分的判断/Filter ==
  In : Inport
  Add : Sum
  Constant : Constant  Value=single(-100)
  Constant1 : Constant  Value=single(100)
  Constant2 : Constant  Value=single(20)
  Constant3 : Constant  Value=single(-20)
  Gain : Gain  Gain=0.5
  Gain1 : Gain  Gain=0.5
  Rate Limiter Dynamic : simulink/Discontinuities/Rate Limiter Dynamic
  Saturation Dynamic : simulink/Discontinuities/Saturation Dynamic  OutMin=[]  OutMax=[]  OutDataTypeStr=Inherit: Same as second input  OutDataType=fixdt(1, 16)  OutScaling=2^-10  DoSatur=off
  Unit Delay : UnitDelay  SampleTime=-1  HasFrameUpgradeWarning=on
  Out : Outport
  wires:
  In/1 -> Saturation Dynamic/2
  Saturation Dynamic/1 -> Rate Limiter Dynamic/2
  Constant1/1 -> Saturation Dynamic/1
  Constant/1 -> Saturation Dynamic/3
  Constant2/1 -> Rate Limiter Dynamic/1
  Constant3/1 -> Rate Limiter Dynamic/3
  Unit Delay/1 -> Gain/1
  Gain/1 -> Add/1
  Add/1 -> Out/1
  Gain1/1 -> Add/2
  Rate Limiter Dynamic/1 -> Gain1/1, Unit Delay/1

== system VxSpdEsti0725/打滑判断/加速度差的微分的判断/Filter1 ==
  In : Inport
  Add : Sum
  Constant : Constant  Value=single(-100)
  Constant1 : Constant  Value=single(100)
  Constant2 : Constant  Value=single(20)
  Constant3 : Constant  Value=single(-20)
  Gain : Gain  Gain=0.5
  Gain1 : Gain  Gain=0.5
  Rate Limiter Dynamic : simulink/Discontinuities/Rate Limiter Dynamic
  Saturation Dynamic : simulink/Discontinuities/Saturation Dynamic  OutMin=[]  OutMax=[]  OutDataTypeStr=Inherit: Same as second input  OutDataType=fixdt(1, 16)  OutScaling=2^-10  DoSatur=off
  Unit Delay : UnitDelay  SampleTime=-1  HasFrameUpgradeWarning=on
  Out : Outport
  wires:
  Rate Limiter Dynamic/1 -> Unit Delay/1, Gain1/1
  Gain1/1 -> Add/2
  Add/1 -> Out/1
  Gain/1 -> Add/1
  Unit Delay/1 -> Gain/1
  Constant3/1 -> Rate Limiter Dynamic/3
  Constant2/1 -> Rate Limiter Dynamic/1
  Constant/1 -> Saturation Dynamic/3
  Constant1/1 -> Saturation Dynamic/1
  Saturation Dynamic/1 -> Rate Limiter Dynamic/2
  In/1 -> Saturation Dynamic/2

== system VxSpdEsti0725/打滑判断/加速度差的微分的判断/Filter2 ==
  In : Inport
  Add : Sum
  Constant : Constant  Value=single(-100)
  Constant1 : Constant  Value=single(100)
  Constant2 : Constant  Value=single(20)
  Constant3 : Constant  Value=single(-20)
  Gain : Gain  Gain=0.5
  Gain1 : Gain  Gain=0.5
  Rate Limiter Dynamic : simulink/Discontinuities/Rate Limiter Dynamic
  Saturation Dynamic : simulink/Discontinuities/Saturation Dynamic  OutMin=[]  OutMax=[]  OutDataTypeStr=Inherit: Same as second input  OutDataType=fixdt(1, 16)  OutScaling=2^-10  DoSatur=off
  Unit Delay : UnitDelay  SampleTime=-1  HasFrameUpgradeWarning=on
  Out : Outport
  wires:
  In/1 -> Saturation Dynamic/2
  Saturation Dynamic/1 -> Rate Limiter Dynamic/2
  Constant1/1 -> Saturation Dynamic/1
  Constant/1 -> Saturation Dynamic/3
  Constant2/1 -> Rate Limiter Dynamic/1
  Constant3/1 -> Rate Limiter Dynamic/3
  Unit Delay/1 -> Gain/1
  Gain/1 -> Add/1
  Add/1 -> Out/1
  Gain1/1 -> Add/2
  Rate Limiter Dynamic/1 -> Gain1/1, Unit Delay/1

== system VxSpdEsti0725/打滑判断/加速度差的微分的判断/Filter3 ==
  In : Inport
  Add : Sum
  Constant : Constant  Value=single(-100)
  Constant1 : Constant  Value=single(100)
  Constant2 : Constant  Value=single(20)
  Constant3 : Constant  Value=single(-20)
  Gain : Gain  Gain=0.5
  Gain1 : Gain  Gain=0.5
  Rate Limiter Dynamic : simulink/Discontinuities/Rate Limiter Dynamic
  Saturation Dynamic : simulink/Discontinuities/Saturation Dynamic  OutMin=[]  OutMax=[]  OutDataTypeStr=Inherit: Same as second input  OutDataType=fixdt(1, 16)  OutScaling=2^-10  DoSatur=off
  Unit Delay : UnitDelay  SampleTime=-1  HasFrameUpgradeWarning=on
  Out : Outport
  wires:
  Rate Limiter Dynamic/1 -> Unit Delay/1, Gain1/1
  Gain1/1 -> Add/2
  Add/1 -> Out/1
  Gain/1 -> Add/1
  Unit Delay/1 -> Gain/1
  Constant3/1 -> Rate Limiter Dynamic/3
  Constant2/1 -> Rate Limiter Dynamic/1
  Constant/1 -> Saturation Dynamic/3
  Constant1/1 -> Saturation Dynamic/1
  Saturation Dynamic/1 -> Rate Limiter Dynamic/2
  In/1 -> Saturation Dynamic/2

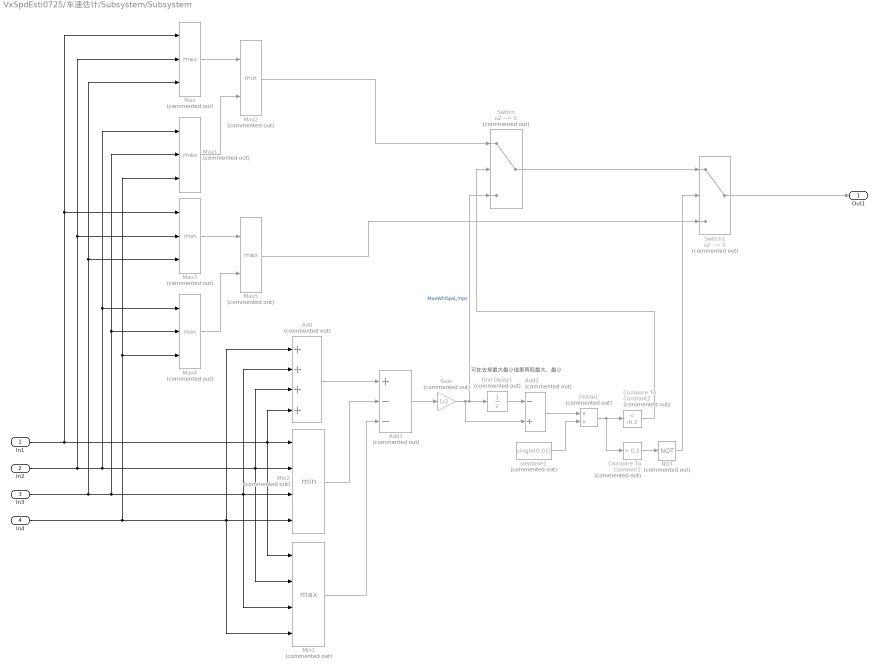
== system VxSpdEsti0725/车速估计/Subsystem/Subsystem ==
  note: 可在去掉最大最小值里再取最大、最小
  In1 : Inport
  In2 : Inport  Port=2
  In3 : Inport  Port=3
  In4 : Inport  Port=4
  Add : Sum  Commented=on  Inputs=++++
  Add1 : Sum  Commented=on  Inputs=+--
  Add2 : Sum  Commented=on  Inputs=-+
  Compare To Constant1 : simulink/Logic and Bit Operations/Compare To Constant  Commented=on  relop=>  const=0.2  OutDataTypeStr=boolean
  Compare To Constant2 : simulink/Logic and Bit Operations/Compare To Constant  Commented=on  relop=<  const=-0.2  OutDataTypeStr=boolean
  Divide1 : Product  Commented=on  Inputs=*/
  Gain : Gain  Commented=on  Gain=1/2
  Max : MinMax  Commented=on  Function=max  Inputs=3
  Max1 : MinMax  Commented=on  Function=max  Inputs=3
  Max2 : MinMax  Commented=on  Inputs=2
  Max3 : MinMax  Commented=on  Inputs=3
  Max4 : MinMax  Commented=on  Inputs=3
  Max5 : MinMax  Commented=on  Function=max  Inputs=2
  Min1 : MinMax  Commented=on  Function=max  Inputs=4
  Min2 : MinMax  Commented=on  Inputs=4
  NOT : Logic  Commented=on  Operator=NOT  AllPortsSameDT=off  OutDataTypeStr=boolean
  Switch : Switch  Commented=on  Criteria=u2 ~= 0  SaturateOnIntegerOverflow=off  InputSameDT=off
  Switch1 : Switch  Commented=on  Criteria=u2 ~= 0  SaturateOnIntegerOverflow=off  InputSameDT=off
  Unit Delay1 : UnitDelay  Commented=on  SampleTime=-1  HasFrameUpgradeWarning=on
  steptime1 : Constant  Commented=on  Value=single(0.01)
  Out1 : Outport
  wires:
  Gain/1 -> Switch/3, Unit Delay1/1, Add2/2  "MaxWhlSpd_mps"
  Add2/1 -> Divide1/1
  In1/1 -> Max/1, Max3/1, Add/4, Min1/1, Min2/1
  In4/1 -> Max1/3, Max4/3, Add/1, Min1/4, Min2/4
  In2/1 -> Max/2, Max3/2, Max1/1, Max4/1, Add/3, Min1/2, Min2/2
  In3/1 -> Max/3, Max3/3, Add/2, Min1/3, Min2/3, Max1/2, Max4/2
  Max5/1 -> Switch1/3
  Unit Delay1/1 -> Add2/1
  Max4/1 -> Max5/2
  Compare To Constant2/1 -> Switch/2
  Max3/1 -> Max5/1
  steptime1/1 -> Divide1/2
  Add/1 -> Add1/1
  Compare To Constant1/1 -> NOT/1
  Divide1/1 -> Compare To Constant1/1, Compare To Constant2/1
  Min2/1 -> Add1/2
  Switch1/1 -> Out1/1
  Add1/1 -> Gain/1
  NOT/1 -> Switch1/2
  Max2/1 -> Switch/1
  Max/1 -> Max2/1
  Max1/1 -> Max2/2
  Switch/1 -> Switch1/1
  Min1/1 -> Add1/3
